simulink model "svpwm_3Level1Phase"  (R2025a)
settings: Solver=ode45  StartTime=0.0  StopTime=0.2  MaxStep=1/100e3/100  MinStep=1/100e3/200  RelTol=1e-3
libraries: spsMosfetLib x14, dspfdesign x9, spsSeriesRLCBranchLib x6, spsVoltageMeasurementLib x5, spsDiodeLib x4, spsCurrentMeasurementLib x3, spsDCVoltageSourceLib x1, simulink x1, sps_lib x1
settings Model: Creator=WYY  LastModifiedBy=jicai
settings SolverCC: AlgebraicLoopSolver=TrustRegion
settings DataIOCC: ReturnWorkspaceOutputs=off
settings DebuggingCC: UnconnectedInputMsg=warning  UnconnectedOutputMsg=warning  UnconnectedLineMsg=warning  ArithmeticOperatorsInVariantConditions=warning
settings ModelReferenceCC: EnableRefExpFcnMdlSchedulingChecks=on
settings SFSimCC: SimUseLocalCustomCode=off  CustomCodeUndefinedFunction=UseInterfaceOnly
settings RTWCC: RTWUseLocalCustomCode=off  GPUComputeCapability=3.5
settings CodeAppCC: StateflowObjectComments=on
settings SimscapeCC: SimscapeNormalizeSystem=off

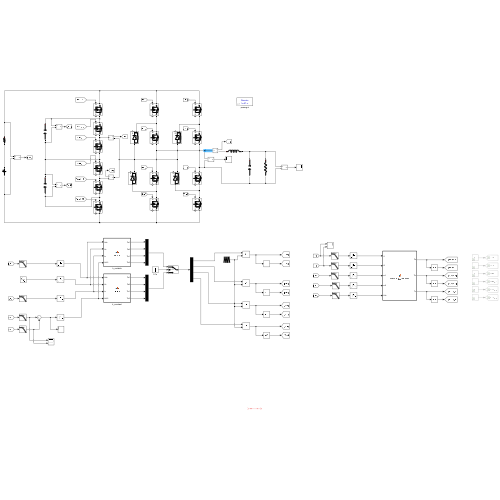
[thumbnail: Simulink's stored preview of the top-level diagram]
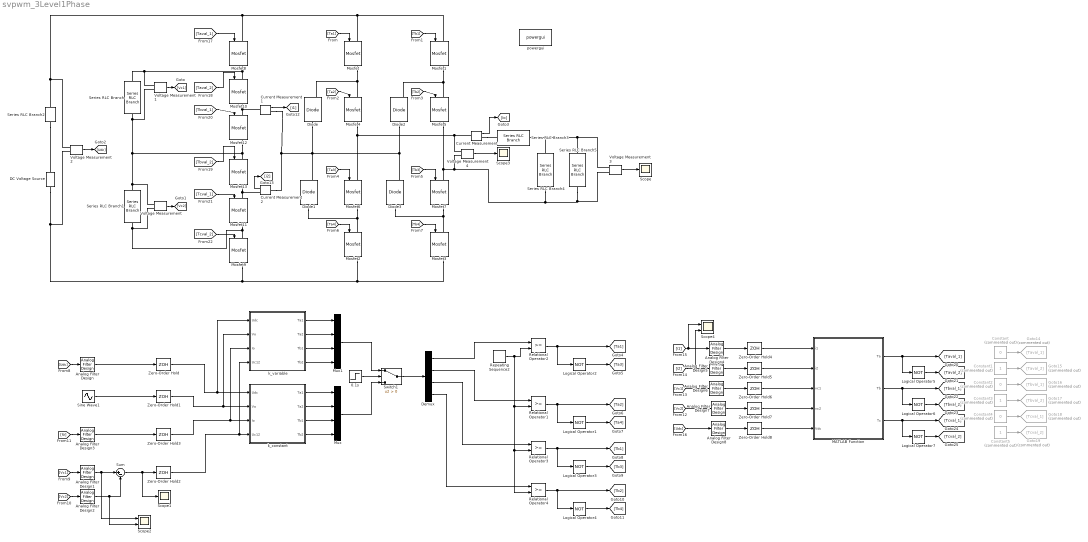
== system svpwm_3Level1Phase ==
  0.1s : Step  Time=0.2  SampleTime=0
  Analog Filter Design{,3..8} (7 alike) : dspfdesign/Analog Filter Design  method=Butterworth  filttype=Lowpass  N=2  Wlo=2*pi*1e3  Whi=80  Rp=2  Rs=40
  Analog Filter Design1 : dspfdesign/Analog Filter Design  method=Butterworth  filttype=Lowpass  N=2  Wlo=2*pi*10e3  Whi=80  Rp=2  Rs=40
  Analog Filter Design2 : dspfdesign/Analog Filter Design  method=Butterworth  filttype=Lowpass  N=2  Wlo=2*pi*10e3  Whi=80  Rp=2  Rs=40
  Constant : Constant  Commented=on  Value=0
  Constant1 : Constant  Commented=on
  Constant2 : Constant  Commented=on  Value=0
  Constant3 : Constant  Commented=on
  Constant4 : Constant  Commented=on  Value=0
  Constant5 : Constant  Commented=on
  Current Measurement : spsCurrentMeasurementLib/Current Measurement  PhasorSimulation=off  OutputType=Complex  PSBequivalent=0
  Current Measurement1 : spsCurrentMeasurementLib/Current Measurement  PhasorSimulation=off  OutputType=Complex  PSBequivalent=0
  Current Measurement2 : spsCurrentMeasurementLib/Current Measurement  PhasorSimulation=off  OutputType=Complex  PSBequivalent=0
  DC Voltage Source : spsDCVoltageSourceLib/DC Voltage Source  Amplitude=400  Measurements=None
  Demux : Demux
  Diode{,1..3} (4 alike) : spsDiodeLib/Diode  Ron=0.001  Lon=0  Vf=0.8  IC=0  UseSnubber=0  Rs=500  Cs=250e-9  Measurements=on
  Goto14 : Goto  Commented=on  GotoTag=Taval_1
  Goto15 : Goto  Commented=on  GotoTag=Taval_2
  Goto16 : Goto  Commented=on  GotoTag=Tbval_1
  Goto17 : Goto  Commented=on  GotoTag=Tbval_2
  Goto18 : Goto  Commented=on  GotoTag=Tcval_1
  Goto19 : Goto  Commented=on  GotoTag=Tcval_2
  Logical Operator{1..7} (7 alike) : Logic  Operator=NOT  AllPortsSameDT=off  OutDataTypeStr=boolean
  MATLAB Function : MATLAB Function  TreatAsAtomicUnit=on
  Mosfet{,1..13} (14 alike) : spsMosfetLib/Mosfet  Ron=0.1  Lon=0  Rd=0.01  Vfd=0  IC=0  Rs=1e5  Cs=inf  Measurements=on
  Mux : Mux
  Mux1 : Mux
  Relational Operator{1..4} (4 alike) : RelationalOperator  OutDataTypeStr=boolean  RndMeth=Simplest  InputSameDT=off
  Repeating Sequence2 : simulink/Sources/Repeating Sequence  rep_seq_t=[0 1/100e3/2 1/100e3]  rep_seq_y=[0.01 0.99 0.01]
  Scope : Scope
      settings: ActiveDisplayYMinimum=-385.78427901086286  ActiveDisplayYMaximum=419.08315334932496
  Scope1 : Scope
      settings: ActiveDisplayYMinimum=-4.7231788824178516  ActiveDisplayYMaximum=76.032530001662565
  Scope2 : Scope  NumInputPorts=2
      settings: ActiveDisplayYMinimum=-12.164414686695521  ActiveDisplayYMaximum=109.47973218025972  DataLoggingVariableName=ScopeData3
  Scope3 : Scope
      settings: ActiveDisplayYMinimum=404.52331193654425  ActiveDisplayYMaximum=435.5661177792087  DataLoggingVariableName=ScopeData2
  Scope4 : Scope  NumInputPorts=2
      settings: ActiveDisplayYMinimum=-19.357294872555265  ActiveDisplayYMaximum=346.96364507181  DataLoggingVariableName=ScopeData4
  Series RLC Branch : spsSeriesRLCBranchLib/Series RLC Branch  LConnTagsString=__new0  RConnTagsString=__new0  BranchType=C  Resistance=1  Inductance=1e-3  SetiL0=off  InitialCurrent=0  Capacitance=300e-6  Setx0=on  InitialVoltage=200  Measurements=None
  Series RLC Branch1 : spsSeriesRLCBranchLib/Series RLC Branch  LConnTagsString=__new0  RConnTagsString=__new0  BranchType=C  Resistance=1  Inductance=1e-3  SetiL0=off  InitialCurrent=0  Capacitance=300e-6  Setx0=on  InitialVoltage=200  Measurements=None
  Series RLC Branch2 : spsSeriesRLCBranchLib/Series RLC Branch  LConnTagsString=__new0  RConnTagsString=__new0  BranchType=R  Resistance=1  Inductance=1e-3  SetiL0=off  InitialCurrent=0  Capacitance=1e-6  Setx0=off  InitialVoltage=0  Measurements=None
  Series RLC Branch3 : spsSeriesRLCBranchLib/Series RLC Branch  LConnTagsString=__new0  RConnTagsString=__new0  BranchType=L  Resistance=1  Inductance=16e-6  SetiL0=off  InitialCurrent=0  Capacitance=1e-6  Setx0=off  InitialVoltage=0  Measurements=None
  Series RLC Branch4 : spsSeriesRLCBranchLib/Series RLC Branch  LConnTagsString=__new0  RConnTagsString=__new0  BranchType=C  Resistance=1  Inductance=1e-3  SetiL0=off  InitialCurrent=0  Capacitance=16e-6  Setx0=off  InitialVoltage=0  Measurements=None
  Series RLC Branch5 : spsSeriesRLCBranchLib/Series RLC Branch  LConnTagsString=__new0  RConnTagsString=__new0  BranchType=R  Resistance=100  Inductance=1e-3  SetiL0=off  InitialCurrent=0  Capacitance=1e-6  Setx0=off  InitialVoltage=0  Measurements=None
  Sine Wave1 : Sin  Amplitude=300  Frequency=2*pi*200  SampleTime=0
  Sum : Sum  Inputs=|+-
  Switch1 : Switch  Criteria=u2 > Threshold  SaturateOnIntegerOverflow=off  InputSameDT=off
  Voltage Measurement{,1..4} (5 alike) : spsVoltageMeasurementLib/Voltage Measurement  PhasorSimulation=off  OutputType=Complex  PSBequivalent=0
  Zero-Order Hold{,1..8} (9 alike) : ZeroOrderHold  SampleTime=1/100e3
  k_constant : MATLAB Function  TreatAsAtomicUnit=on
  k_variable : MATLAB Function  TreatAsAtomicUnit=on
  powergui : sps_lib/powergui  Priority=1  SimulationMode=Discrete  SampleTime=1e-7  frequency=60  Iterations=50  frequencyindice=0  Pbase=100e6  ErrMax=1e-4  UnitsV=kV  UnitsW=MW  buscounter=0  FunctionMessages=off  echomessages=off  EnableUseOfTLC=off  CurrentSourceSwitches=off  DisableSnubberDevices=off  DisableRonSwitches=off  DisableVfSwitches=off  DisplayEquations=off  AutomaticDiscreteSolvers=off  SolverType=Tustin/Backward Euler (TBE)  Interpol=off  ExternalGateDelay=off  methode=off  Ts=100  x0status=blocks  SPID=on  SwTol=0  HookPort=off  NonlinearTolerance=1e-4  nMaxIteration=100  ContinueOnMaxIteration=off  RestoreLinks=warning  ResistiveCurrentMeasurement=off  Frange=[0:2:500]  Ylog=off  Xlog=on  ShowGrid=off  save=off  variable=ZData  structure=0  ZoomFFT=off  StartTime=0.0  cycles=1  DisplayStyle=1  fundamental=60  FreqAxis=off  MaxFrequency=1000  frequencyindicesteady=1  RmsSteady=1  display=off
  wires:
  [Ta1] -> Mosfet/1
  [Tb1] -> Mosfet1/1
  [Ta2] -> Mosfet4/1
  [Tb2] -> Mosfet5/1
  [Ta3] -> Mosfet6/1
  [Ta4] -> Mosfet2/1
  [Tb4] -> Mosfet3/1
  [Tb3] -> Mosfet7/1
  Voltage Measurement1/1 -> [Vc1]
  Voltage Measurement/1 -> [Vc2]
  Voltage Measurement2/1 -> [Udc]
  Current Measurement/1 -> [Io]
  [Udc] -> Analog Filter Design/1
  [Vc1] -> Analog Filter Design1/1
  [Vc2] -> Analog Filter Design2/1
  [Io] -> Analog Filter Design3/1
  Analog Filter Design1/1 -> Scope2/1, Sum/1
  Analog Filter Design2/1 -> Scope2/2, Sum/2
  Analog Filter Design/1 -> Zero-Order Hold/1
  Sum/1 -> Scope1/1, Zero-Order Hold2/1
  Analog Filter Design3/1 -> Zero-Order Hold3/1
  Zero-Order Hold/1 -> k_variable/1(Udc), k_constant/1(Udc)
  Zero-Order Hold1/1 -> k_variable/2(Vo), k_constant/2(Vo)
  Zero-Order Hold3/1 -> k_constant/3(Io), k_variable/3(Io)
  Zero-Order Hold2/1 -> k_variable/4(Uc12), k_constant/4(Uc12)
  Repeating Sequence2/1 -> Relational Operator4/2, Relational Operator3/2, Relational Operator1/2, Relational Operator2/2
  Relational Operator2/1 -> Logical Operator2/1, [Ta1]
  Logical Operator2/1 -> [Ta3]
  Logical Operator1/1 -> [Ta4]
  Relational Operator1/1 -> [Ta2], Logical Operator1/1
  Relational Operator3/1 -> Logical Operator3/1, [Tb1]
  Logical Operator3/1 -> [Tb3]
  Logical Operator4/1 -> [Tb4]
  Relational Operator4/1 -> [Tb2], Logical Operator4/1
  Voltage Measurement3/1 -> Scope/1
  Voltage Measurement4/1 -> Scope3/1
  k_constant/2(Ta2) -> Mux/2
  k_constant/3(Tb1) -> Mux/3
  k_constant/4(Tb2) -> Mux/4
  k_constant/1(Ta1) -> Mux/1
  k_variable/1(Ta1) -> Mux1/1
  k_variable/2(Ta2) -> Mux1/2
  k_variable/3(Tb1) -> Mux1/3
  k_variable/4(Tb2) -> Mux1/4
  0.1s/1 -> Switch1/2
  Mux1/1 -> Switch1/1
  Mux/1 -> Switch1/3
  Switch1/1 -> Demux/1
  Demux/1 -> Relational Operator2/1
  Demux/2 -> Relational Operator1/1
  Demux/3 -> Relational Operator3/1
  Demux/4 -> Relational Operator4/1
  Sine Wave1/1 -> Zero-Order Hold1/1
  Current Measurement1/1 -> [i1]
  MATLAB Function/1(Ta) -> [Taval_1], Logical Operator5/1
  Logical Operator5/1 -> [Taval_2]
  Logical Operator6/1 -> [Tbval_2]
  MATLAB Function/2(Tb) -> [Tbval_1], Logical Operator6/1
  MATLAB Function/3(Tc) -> [Tcval_1], Logical Operator7/1
  Logical Operator7/1 -> [Tcval_2]
  [Taval_1] -> Mosfet8/1
  [Taval_2] -> Mosfet10/1
  [Tbval_2] -> Mosfet13/1
  [Tbval_1] -> Mosfet12/1
  [Tcval_1] -> Mosfet11/1
  [Tcval_2] -> Mosfet9/1
  ? -> ?
  [i1] -> Scope4/1, Analog Filter Design4/1
  Analog Filter Design4/1 -> Zero-Order Hold4/1
  Zero-Order Hold4/1 -> MATLAB Function/1(i1)
  Zero-Order Hold5/1 -> MATLAB Function/2(i2)
  Analog Filter Design5/1 -> Zero-Order Hold5/1
  [i2] -> Scope4/2, Analog Filter Design5/1
  Analog Filter Design6/1 -> Zero-Order Hold6/1
  Zero-Order Hold7/1 -> MATLAB Function/4(vc2)
  Analog Filter Design7/1 -> Zero-Order Hold7/1
  Zero-Order Hold6/1 -> MATLAB Function/3(vc1)
  [Vc1] -> Analog Filter Design6/1
  [Vc2] -> Analog Filter Design7/1
  [Udc] -> Analog Filter Design8/1
  Analog Filter Design8/1 -> Zero-Order Hold8/1
  Zero-Order Hold8/1 -> MATLAB Function/5(Vdc)
  Constant/1 -> Goto14/1
  Constant2/1 -> Goto16/1
  Constant4/1 -> Goto18/1
  Constant1/1 -> Goto15/1
  Constant3/1 -> Goto17/1
  Constant5/1 -> Goto19/1
  Current Measurement2/1 -> [i2]
  connections:
  Series RLC Branch2/RConn1 -- DC Voltage Source/RConn1
  Mosfet/RConn1 -- Mosfet4/LConn1 -- Diode/RConn1
  Mosfet1/RConn1 -- Mosfet5/LConn1 -- Diode2/RConn1
  Mosfet4/RConn1 -- Voltage Measurement4/LConn1 -- Current Measurement/LConn1 -- Mosfet6/LConn1
  Mosfet5/RConn1 -- Voltage Measurement4/LConn2 -- Voltage Measurement3/LConn2 -- Series RLC Branch5/RConn1 -- Series RLC Branch4/RConn1 -- Mosfet7/LConn1
  Mosfet6/RConn1 -- Diode1/LConn1 -- Mosfet2/LConn1
  Mosfet7/RConn1 -- Mosfet3/LConn1 -- Diode3/LConn1
  Series RLC Branch4/LConn1 -- Voltage Measurement3/LConn1 -- Series RLC Branch5/LConn1 -- Series RLC Branch3/RConn1
  Current Measurement/RConn1 -- Series RLC Branch3/LConn1
  Mosfet10/LConn1 -- Voltage Measurement1/LConn1 -- Series RLC Branch/LConn1 -- Mosfet8/RConn1
  Mosfet11/RConn1 -- Voltage Measurement/LConn2 -- Series RLC Branch1/RConn1 -- Mosfet9/LConn1
  Diode2/LConn1 -- Diode3/RConn1 -- Current Measurement2/LConn1 -- Current Measurement1/RConn1 -- Diode1/RConn1 -- Diode/LConn1
  Mosfet12/LConn1 -- Current Measurement1/LConn1 -- Mosfet10/RConn1
  Mosfet11/LConn1 -- Current Measurement2/RConn1 -- Mosfet13/RConn1
  Mosfet9/RConn1 -- DC Voltage Source/LConn1 -- Voltage Measurement2/LConn2 -- Mosfet2/RConn1 -- Mosfet3/RConn1
  Mosfet8/LConn1 -- Series RLC Branch2/LConn1 -- Voltage Measurement2/LConn1 -- Mosfet/LConn1 -- Mosfet1/LConn1
  Mosfet13/LConn1 -- Mosfet12/RConn1 -- Voltage Measurement1/LConn2 -- Series RLC Branch/RConn1 -- Series RLC Branch1/LConn1 -- Voltage Measurement/LConn1

== matlab function svpwm_3Level1Phase/k_variable ==
  data: Udc input; Ta1 output; Vo input; Io input; Uc12 input; Ta2 output; Tb1 output; Tb2 output
function [Ta1,Ta2,Tb1,Tb2] = svpwm(Udc,Vo,Io,Uc12)
%   判断扇区
k = 0.5;
Tc = 1/(100e3);
m = Vo/(Udc);  
if ( m>=0.5 )&&( m<=1 )
    sector = 1;
elseif ( m>=0 )&&( m<0.5 )
    sector = 2;
elseif ( m>=-0.5 )&&( m<0 )
    sector = 3;
else
    sector = 4;
end

%   通过两个电容之间压差来调整系数k
if ( Io>0 )
    if ( Uc12>0 )
        k = 0.75;
    else
        k = 0.25;
    end
else
    if ( Uc12>0 )
        k = 0.25;
    else
        k = 0.75;
    end
end
%   计算时间
Ta1 = 0;
Ta2 = 0;
Tb1 = 0;
Tb2 = 0;
switch sector
    case 1  %扇区1
        Tl = (2*Vo-Udc)/Udc*Tc;
        Ts = 2*(Udc-Vo)/Udc*Tc;
        Ta1 = (Tl+k*Ts)/Tc;
        Ta2 = 1;
        Tb1 = 0;
        Tb2 = k*Ts/Tc;
    case 2  %扇区2
        Ts = 2*Vo/Udc*Tc;
        To = (Udc-2*Vo)/Udc*Tc;
        Ta1 = k*Ts/Tc;
        Ta2 = 1;
        Tb1 = 0;
        Tb2 = (k*Ts+To)/Tc;
    case 3  %扇区3
        Ts = -2*Vo/Udc*Tc;
        To = (Udc+2*Vo)/Udc*Tc;
        Ta1 = 0;
        Ta2 = ( (1-k)*Ts+To )/Tc;
        Tb1 = (1-k)*Ts/Tc;
        Tb2 = 1;
    case 4  %扇区4
        Tl = -(2*Vo+Udc)/Udc*Tc;
        Ts = 2*(Vo+Udc)/Udc*Tc;
        Ta1 = 0;
        Ta2 = (1-k)*Ts/Tc;
        Tb1 = ( (1-k)*Ts+Tl )/Tc;
        Tb2 = 1;
end

== matlab function svpwm_3Level1Phase/k_constant ==
  data: Udc input; Ta1 output; Vo input; Io input; Uc12 input; Ta2 output; Tb1 output; Tb2 output
function [Ta1,Ta2,Tb1,Tb2] = svpwm(Udc,Vo,Io,Uc12)
%   判断扇区
k = 0.5;
Tc = 1/(100e3);
m = Vo/(Udc);  
if ( m>=0.5 )&&( m<=1 )
    sector = 1;
elseif ( m>=0 )&&( m<0.5 )
    sector = 2;
elseif ( m>=-0.5 )&&( m<0 )
    sector = 3;
else
    sector = 4;
end

%   计算时间
Ta1 = 0;
Ta2 = 0;
Tb1 = 0;
Tb2 = 0;
switch sector
    case 1  %扇区1
        Tl = (2*Vo-Udc)/Udc*Tc;
        Ts = 2*(Udc-Vo)/Udc*Tc;
        Ta1 = (Tl+k*Ts)/Tc;
        Ta2 = 1;
        Tb1 = 0;
        Tb2 = k*Ts/Tc;
    case 2  %扇区2
        Ts = 2*Vo/Udc*Tc;
        To = (Udc-2*Vo)/Udc*Tc;
        Ta1 = k*Ts/Tc;
        Ta2 = 1;
        Tb1 = 0;
        Tb2 = (k*Ts+To)/Tc;
    case 3  %扇区3
        Ts = -2*Vo/Udc*Tc;
        To = (Udc+2*Vo)/Udc*Tc;
        Ta1 = 0;
        Ta2 = ( (1-k)*Ts+To )/Tc;
        Tb1 = (1-k)*Ts/Tc;
        Tb2 = 1;
    case 4  %扇区4
        Tl = -(2*Vo+Udc)/Udc*Tc;
        Ts = 2*(Vo+Udc)/Udc*Tc;
        Ta1 = 0;
        Ta2 = (1-k)*Ts/Tc;
        Tb1 = ( (1-k)*Ts+Tl )/Tc;
        Tb2 = 1;
end

== matlab function svpwm_3Level1Phase/MATLAB Function ==
  data: i1 input; Ta output; i2 input; vc1 input; vc2 input; Vdc input; Tb output; Tc output
function [Ta, Tb, Tc] = balancing_controller(i1, i2, vc1, vc2, Vdc)
% 输入参数：
% i1, i2: 两个钳位点电流 (流入为正)
% vc1, vc2: 两个飞跨电容的实测电压
% Vdc: 直流母线总电压
% Tc: 开关周期 (如 1/100e3)
% 输出参数：
% Ta: 状态 [101010] 的作用时间 (归一化或实际时间)
% Tb: 状态 [010101] 的作用时间

%% 1. 初始化与偏差计算
Vref = Vdc / 2;
dv1 = vc1 - Vref;
dv2 = vc2 - Vref;

% 初始默认使用平衡分配
Ta = 1; 
Tb = 1;
Tc = 1;

%% 2. 区域判断 (基于 i1-i2 坐标系)
% 计算电流向量的角度 (atan2 返回 -pi 到 pi)
theta_rad = atan2(i2, i1);
theta = rad2deg(theta_rad);
if theta < 0
    theta = theta + 360; % 转换为 0-360度
end

% 定义区域 (根据专利描述)
if (theta >= 0 && theta < 90)
    sector = 1;
elseif (theta >= 90 && theta < 135)
    sector = 2;
elseif (theta >= 135 && theta < 180)
    sector = 3;
elseif (theta >= 180 && theta < 270)
    sector = 4;
elseif (theta >= 270 && theta < 315)
    sector = 5;
else % 315 - 360
    sector = 6;
end

%% 3. 优先级决策与开关状态选择
switch sector
    case 1 % i1>0, i2>0, i1+i2>0
        if abs(dv1) >= abs(dv2)
            if dv1 > 0, [Ta, Tb, Tc] = use_101010(); else, [Ta, Tb, Tc] = use_010101(); end
        else
            if dv2 > 0, [Ta, Tb, Tc] = use_101010(); else, [Ta, Tb, Tc] = use_010101(); end
        end
        
    case 2 % i1<0, i2>0, i1+i2>0 (优先调 C2)
        if dv2 > 0, [Ta, Tb, Tc] = use_101010(); else, [Ta, Tb, Tc] = use_010101(); end
        
    case 3 % i1<0, i2<0, i1+i2<0 (优先调 C1)
        if dv1 > 0, [Ta, Tb, Tc] = use_010101(); else, [Ta, Tb, Tc] = use_101010(); end
        
    case 4 % i1<0, i2<0, i1+i2<0 (负向区域，逻辑反向)
        if abs(dv1) >= abs(dv2)
            if dv1 > 0, [Ta, Tb, Tc] = use_010101(); else, [Ta, Tb, Tc] = use_101010(); end
        else
            if dv2 > 0, [Ta, Tb, Tc] = use_010101(); else, [Ta, Tb, Tc] = use_101010(); end
        end
        
    case 5 % i1>0, i2<0, i1+i2<0 (优先调 C2)
        if dv2 > 0, [Ta, Tb, Tc] = use_010101(); else, [Ta, Tb, Tc] = use_101010(); end
        
    case 6 % i1>0, i2<0, i1+i2>0 (优先调 C1)
        if dv1 > 0, [Ta, Tb, Tc] = use_101010(); else, [Ta, Tb, Tc] = use_010101(); end
end

%% 内部辅助函数：定义时间分配倾向
    function [Ta_val, Tb_val, Tc_val] = use_101010()
        Ta_val = 1;
        Tb_val = 1;
        Tc_val = 1;
    end

    function [Ta_val, Tb_val, Tc_val] = use_010101()
        Ta_val = 0;
        Tb_val = 0;
        Tc_val = 0;
    end

end
